simulink model "MyVhclOperator_RTW"  (Simulink 10.3)
settings: Solver=ode1  StartTime=0.0  StopTime=inf  FixedStep=0.001  RelTol=1e-3
PreLoadFcn:
  | vehicle = 'Car'; if ~length(which('cmcmd')), cmenv; end
  | MyVhclOperator_RTW_bus
InitFcn:
  | vehicle = 'Car'; if ~length(which('cmcmd')), cmenv; end
  | MyVhclOperator_RTW_bus
undefined symbols (not defined in the file or in its folder): OperationFinished, Phase, SteerAng, VCBus
libraries: simulink x45
(part 3 of 3)

== system MyVhclOperator_RTW/MyVhclOperator/Trg: OperState_Absent/OperState_Driving/Drive2Off/Wait until Standstill ==
  BusIn : Inport
  Action Port : ActionPort  ActionPortLabel=case: { }
  Bus Assignment : BusAssignment  AssignedSignals=Phase
  Bus Selector : BusSelector  OutputSignals=Velocity
  Compare To Constant : simulink/Logic and Bit Operations/Compare To Constant  SystemSampleTime=-1  relop=<=  const=0.1  LogicOutDataTypeMode=uint8
  Constant : Constant  Value=3
  Constant1 : Constant  Value=2
  Signal Conversion : SignalConversion  ConversionOutput=Bus copy  OverrideOpt=off
  Switch : Switch  Criteria=u2 ~= 0
  BusOut : Outport  InitialOutput=[0]  VectorParamsAs1DForOutWhenUnconnected=off
  wires:
  Bus Assignment/1 -> BusOut/1
  BusIn/1 -> Bus Selector/1, Signal Conversion/1
  Switch/1 -> Bus Assignment/2
  Bus Selector/1 -> Compare To Constant/1  "<Velocity>"
  Constant/1 -> Switch/1
  Constant1/1 -> Switch/3
  Compare To Constant/1 -> Switch/2
  Signal Conversion/1 -> Bus Assignment/1

== system MyVhclOperator_RTW/MyVhclOperator/Trg: OperState_Accessory/OperState_Driving/Drive2Off/Active Brake ==
  BusIn : Inport
  Action Port : ActionPort  ActionPortLabel=case: { }
  Bus Assignment1 : BusAssignment  AssignedSignals=VCBus.Key,VCBus.GearNo,VCBus.SelectorCtrl,VCBus.Gas,VCBus.Clutch,VCBus.Brake,VCBus.BrakePark,Phase
  Bus Selector : BusSelector  OutputSignals=GBKind
  Bus Selector1 : BusSelector  OutputSignals=Key,GearNo,SelectorCtrl,Gas,Clutch,Brake,BrakePark
  Constant : Constant  Value=2
  OperState: Braking : Subsystem
  Signal Conversion : SignalConversion  ConversionOutput=Bus copy  OverrideOpt=off
  BusOut : Outport  InitialOutput=[0]  VectorParamsAs1DForOutWhenUnconnected=off
  wires:
  BusIn/1 -> Bus Selector/1, Signal Conversion/1
  Bus Selector/1 -> OperState: Braking/1(GBKind)  "<GBKind>"
  OperState: Braking/1(BusOut) -> Bus Selector1/1  "VC_Bus"
  Constant/1 -> Bus Assignment1/9
  Bus Assignment1/1 -> BusOut/1
  Signal Conversion/1 -> Bus Assignment1/1
  Bus Selector1/1 -> Bus Assignment1/2  "<Key>"
  Bus Selector1/2 -> Bus Assignment1/3  "<GearNo>"
  Bus Selector1/3 -> Bus Assignment1/4  "<SelectorCtrl>"
  Bus Selector1/4 -> Bus Assignment1/5  "<Gas>"
  Bus Selector1/5 -> Bus Assignment1/6  "<Clutch>"
  Bus Selector1/6 -> Bus Assignment1/7  "<Brake>"
  Bus Selector1/7 -> Bus Assignment1/8  "<BrakePark>"

== system MyVhclOperator_RTW/MyVhclOperator/Trg: OperState_Accessory/OperState_Driving/Drive2Off/Brake to standstill? ==
  BusIn : Inport
  Action Port : ActionPort  ActionPortLabel=case: { }
  Bus Assignment : BusAssignment  AssignedSignals=Phase
  Bus Selector : BusSelector  OutputSignals=Velocity
  Compare To Constant : simulink/Logic and Bit Operations/Compare To Constant  SystemSampleTime=-1  relop=>  const=0.1  LogicOutDataTypeMode=uint8
  Constant : Constant
  Constant1 : Constant  Value=3
  Signal Conversion : SignalConversion  ConversionOutput=Bus copy  OverrideOpt=off
  Switch : Switch  Criteria=u2 ~= 0
  BusOut : Outport  InitialOutput=[0]  VectorParamsAs1DForOutWhenUnconnected=off
  wires:
  Bus Assignment/1 -> BusOut/1
  BusIn/1 -> Bus Selector/1, Signal Conversion/1
  Switch/1 -> Bus Assignment/2
  Bus Selector/1 -> Compare To Constant/1  "<Velocity>"
  Constant/1 -> Switch/1
  Constant1/1 -> Switch/3
  Compare To Constant/1 -> Switch/2
  Signal Conversion/1 -> Bus Assignment/1

== system MyVhclOperator_RTW/MyVhclOperator/Trg: OperState_Accessory/OperState_Driving/Drive2Off/Key PowerOff ==
  BusIn : Inport
  Action Port : ActionPort  ActionPortLabel=case: { }
  Bus Assignment : BusAssignment  AssignedSignals=VCBus.Key,SteerAng,Phase
  Constant : Constant  Value=4
  Constant2 : Constant  Value=0.0
  KeyPos_KeyIn_PowerOff : Constant
  Signal Conversion : SignalConversion  ConversionOutput=Bus copy  OverrideOpt=off
  BusOut : Outport  InitialOutput=[0]  VectorParamsAs1DForOutWhenUnconnected=off
  wires:
  BusIn/1 -> Signal Conversion/1
  Bus Assignment/1 -> BusOut/1
  Constant/1 -> Bus Assignment/4
  Constant2/1 -> Bus Assignment/3
  KeyPos_KeyIn_PowerOff/1 -> Bus Assignment/2
  Signal Conversion/1 -> Bus Assignment/1

== system MyVhclOperator_RTW/MyVhclOperator/Trg: OperState_Accessory/OperState_Driving/Drive2Off/Wait for PowerOff ==
  BusIn : Inport
  Action Port : ActionPort  ActionPortLabel=case: { }
  Signal Conversion : SignalConversion  ConversionOutput=Bus copy  OverrideOpt=off
  BusOut : Outport  VectorParamsAs1DForOutWhenUnconnected=off
  wires:
  BusIn/1 -> Signal Conversion/1
  Signal Conversion/1 -> BusOut/1

== system MyVhclOperator_RTW/MyVhclOperator/Trg: OperState_Accessory/OperState_Driving/Drive2Off/Wait until Standstill ==
  BusIn : Inport
  Action Port : ActionPort  ActionPortLabel=case: { }
  Bus Assignment : BusAssignment  AssignedSignals=Phase
  Bus Selector : BusSelector  OutputSignals=Velocity
  Compare To Constant : simulink/Logic and Bit Operations/Compare To Constant  SystemSampleTime=-1  relop=<=  const=0.1  LogicOutDataTypeMode=uint8
  Constant : Constant  Value=3
  Constant1 : Constant  Value=2
  Signal Conversion : SignalConversion  ConversionOutput=Bus copy  OverrideOpt=off
  Switch : Switch  Criteria=u2 ~= 0
  BusOut : Outport  InitialOutput=[0]  VectorParamsAs1DForOutWhenUnconnected=off
  wires:
  Bus Assignment/1 -> BusOut/1
  BusIn/1 -> Bus Selector/1, Signal Conversion/1
  Switch/1 -> Bus Assignment/2
  Bus Selector/1 -> Compare To Constant/1  "<Velocity>"
  Constant/1 -> Switch/1
  Constant1/1 -> Switch/3
  Compare To Constant/1 -> Switch/2
  Signal Conversion/1 -> Bus Assignment/1

== system MyVhclOperator_RTW/MyVhclOperator/Trg: OperState_PowerOff/OperState_Driving/Drive2Off/Active Brake ==
  BusIn : Inport
  Action Port : ActionPort  ActionPortLabel=case: { }
  Bus Assignment1 : BusAssignment  AssignedSignals=VCBus.Key,VCBus.GearNo,VCBus.SelectorCtrl,VCBus.Gas,VCBus.Clutch,VCBus.Brake,VCBus.BrakePark,Phase
  Bus Selector : BusSelector  OutputSignals=GBKind
  Bus Selector1 : BusSelector  OutputSignals=Key,GearNo,SelectorCtrl,Gas,Clutch,Brake,BrakePark
  Constant : Constant  Value=2
  OperState: Braking : Subsystem
  Signal Conversion : SignalConversion  ConversionOutput=Bus copy  OverrideOpt=off
  BusOut : Outport  InitialOutput=[0]  VectorParamsAs1DForOutWhenUnconnected=off
  wires:
  BusIn/1 -> Bus Selector/1, Signal Conversion/1
  Bus Selector/1 -> OperState: Braking/1(GBKind)  "<GBKind>"
  OperState: Braking/1(BusOut) -> Bus Selector1/1  "VC_Bus"
  Constant/1 -> Bus Assignment1/9
  Bus Assignment1/1 -> BusOut/1
  Signal Conversion/1 -> Bus Assignment1/1
  Bus Selector1/1 -> Bus Assignment1/2  "<Key>"
  Bus Selector1/2 -> Bus Assignment1/3  "<GearNo>"
  Bus Selector1/3 -> Bus Assignment1/4  "<SelectorCtrl>"
  Bus Selector1/4 -> Bus Assignment1/5  "<Gas>"
  Bus Selector1/5 -> Bus Assignment1/6  "<Clutch>"
  Bus Selector1/6 -> Bus Assignment1/7  "<Brake>"
  Bus Selector1/7 -> Bus Assignment1/8  "<BrakePark>"

== system MyVhclOperator_RTW/MyVhclOperator/Trg: OperState_PowerOff/OperState_Driving/Drive2Off/Brake to standstill? ==
  BusIn : Inport
  Action Port : ActionPort  ActionPortLabel=case: { }
  Bus Assignment : BusAssignment  AssignedSignals=Phase
  Bus Selector : BusSelector  OutputSignals=Velocity
  Compare To Constant : simulink/Logic and Bit Operations/Compare To Constant  SystemSampleTime=-1  relop=>  const=0.1  LogicOutDataTypeMode=uint8
  Constant : Constant
  Constant1 : Constant  Value=3
  Signal Conversion : SignalConversion  ConversionOutput=Bus copy  OverrideOpt=off
  Switch : Switch  Criteria=u2 ~= 0
  BusOut : Outport  InitialOutput=[0]  VectorParamsAs1DForOutWhenUnconnected=off
  wires:
  Bus Assignment/1 -> BusOut/1
  BusIn/1 -> Bus Selector/1, Signal Conversion/1
  Switch/1 -> Bus Assignment/2
  Bus Selector/1 -> Compare To Constant/1  "<Velocity>"
  Constant/1 -> Switch/1
  Constant1/1 -> Switch/3
  Compare To Constant/1 -> Switch/2
  Signal Conversion/1 -> Bus Assignment/1

== system MyVhclOperator_RTW/MyVhclOperator/Trg: OperState_PowerOff/OperState_Driving/Drive2Off/Key PowerOff ==
  BusIn : Inport
  Action Port : ActionPort  ActionPortLabel=case: { }
  Bus Assignment : BusAssignment  AssignedSignals=VCBus.Key,SteerAng,Phase
  Constant : Constant  Value=4
  Constant2 : Constant  Value=0.0
  KeyPos_KeyIn_PowerOff : Constant
  Signal Conversion : SignalConversion  ConversionOutput=Bus copy  OverrideOpt=off
  BusOut : Outport  InitialOutput=[0]  VectorParamsAs1DForOutWhenUnconnected=off
  wires:
  BusIn/1 -> Signal Conversion/1
  Bus Assignment/1 -> BusOut/1
  Constant/1 -> Bus Assignment/4
  Constant2/1 -> Bus Assignment/3
  KeyPos_KeyIn_PowerOff/1 -> Bus Assignment/2
  Signal Conversion/1 -> Bus Assignment/1

== system MyVhclOperator_RTW/MyVhclOperator/Trg: OperState_PowerOff/OperState_Driving/Drive2Off/Wait for PowerOff ==
  BusIn : Inport
  Action Port : ActionPort  ActionPortLabel=case: { }
  Signal Conversion : SignalConversion  ConversionOutput=Bus copy  OverrideOpt=off
  BusOut : Outport  VectorParamsAs1DForOutWhenUnconnected=off
  wires:
  BusIn/1 -> Signal Conversion/1
  Signal Conversion/1 -> BusOut/1

== system MyVhclOperator_RTW/MyVhclOperator/Trg: OperState_PowerOff/OperState_Driving/Drive2Off/Wait until Standstill ==
  BusIn : Inport
  Action Port : ActionPort  ActionPortLabel=case: { }
  Bus Assignment : BusAssignment  AssignedSignals=Phase
  Bus Selector : BusSelector  OutputSignals=Velocity
  Compare To Constant : simulink/Logic and Bit Operations/Compare To Constant  SystemSampleTime=-1  relop=<=  const=0.1  LogicOutDataTypeMode=uint8
  Constant : Constant  Value=3
  Constant1 : Constant  Value=2
  Signal Conversion : SignalConversion  ConversionOutput=Bus copy  OverrideOpt=off
  Switch : Switch  Criteria=u2 ~= 0
  BusOut : Outport  InitialOutput=[0]  VectorParamsAs1DForOutWhenUnconnected=off
  wires:
  Bus Assignment/1 -> BusOut/1
  BusIn/1 -> Bus Selector/1, Signal Conversion/1
  Switch/1 -> Bus Assignment/2
  Bus Selector/1 -> Compare To Constant/1  "<Velocity>"
  Constant/1 -> Switch/1
  Constant1/1 -> Switch/3
  Compare To Constant/1 -> Switch/2
  Signal Conversion/1 -> Bus Assignment/1

== system MyVhclOperator_RTW/MyVhclOperator/Trg: OperState_PowerOn/OperState_Driving/Drive2Off/Active Brake ==
  BusIn : Inport
  Action Port : ActionPort  ActionPortLabel=case: { }
  Bus Assignment1 : BusAssignment  AssignedSignals=VCBus.Key,VCBus.GearNo,VCBus.SelectorCtrl,VCBus.Gas,VCBus.Clutch,VCBus.Brake,VCBus.BrakePark,Phase
  Bus Selector : BusSelector  OutputSignals=GBKind
  Bus Selector1 : BusSelector  OutputSignals=Key,GearNo,SelectorCtrl,Gas,Clutch,Brake,BrakePark
  Constant : Constant  Value=2
  OperState: Braking : Subsystem
  Signal Conversion : SignalConversion  ConversionOutput=Bus copy  OverrideOpt=off
  BusOut : Outport  InitialOutput=[0]  VectorParamsAs1DForOutWhenUnconnected=off
  wires:
  BusIn/1 -> Bus Selector/1, Signal Conversion/1
  Bus Selector/1 -> OperState: Braking/1(GBKind)  "<GBKind>"
  OperState: Braking/1(BusOut) -> Bus Selector1/1  "VC_Bus"
  Constant/1 -> Bus Assignment1/9
  Bus Assignment1/1 -> BusOut/1
  Signal Conversion/1 -> Bus Assignment1/1
  Bus Selector1/1 -> Bus Assignment1/2  "<Key>"
  Bus Selector1/2 -> Bus Assignment1/3  "<GearNo>"
  Bus Selector1/3 -> Bus Assignment1/4  "<SelectorCtrl>"
  Bus Selector1/4 -> Bus Assignment1/5  "<Gas>"
  Bus Selector1/5 -> Bus Assignment1/6  "<Clutch>"
  Bus Selector1/6 -> Bus Assignment1/7  "<Brake>"
  Bus Selector1/7 -> Bus Assignment1/8  "<BrakePark>"

== system MyVhclOperator_RTW/MyVhclOperator/Trg: OperState_PowerOn/OperState_Driving/Drive2Off/Brake to standstill? ==
  BusIn : Inport
  Action Port : ActionPort  ActionPortLabel=case: { }
  Bus Assignment : BusAssignment  AssignedSignals=Phase
  Bus Selector : BusSelector  OutputSignals=Velocity
  Compare To Constant : simulink/Logic and Bit Operations/Compare To Constant  SystemSampleTime=-1  relop=>  const=0.1  LogicOutDataTypeMode=uint8
  Constant : Constant
  Constant1 : Constant  Value=3
  Signal Conversion : SignalConversion  ConversionOutput=Bus copy  OverrideOpt=off
  Switch : Switch  Criteria=u2 ~= 0
  BusOut : Outport  InitialOutput=[0]  VectorParamsAs1DForOutWhenUnconnected=off
  wires:
  Bus Assignment/1 -> BusOut/1
  BusIn/1 -> Bus Selector/1, Signal Conversion/1
  Switch/1 -> Bus Assignment/2
  Bus Selector/1 -> Compare To Constant/1  "<Velocity>"
  Constant/1 -> Switch/1
  Constant1/1 -> Switch/3
  Compare To Constant/1 -> Switch/2
  Signal Conversion/1 -> Bus Assignment/1

== system MyVhclOperator_RTW/MyVhclOperator/Trg: OperState_PowerOn/OperState_Driving/Drive2Off/Key PowerOff ==
  BusIn : Inport
  Action Port : ActionPort  ActionPortLabel=case: { }
  Bus Assignment : BusAssignment  AssignedSignals=VCBus.Key,SteerAng,Phase
  Constant : Constant  Value=4
  Constant2 : Constant  Value=0.0
  KeyPos_KeyIn_PowerOff : Constant
  Signal Conversion : SignalConversion  ConversionOutput=Bus copy  OverrideOpt=off
  BusOut : Outport  InitialOutput=[0]  VectorParamsAs1DForOutWhenUnconnected=off
  wires:
  BusIn/1 -> Signal Conversion/1
  Bus Assignment/1 -> BusOut/1
  Constant/1 -> Bus Assignment/4
  Constant2/1 -> Bus Assignment/3
  KeyPos_KeyIn_PowerOff/1 -> Bus Assignment/2
  Signal Conversion/1 -> Bus Assignment/1

== system MyVhclOperator_RTW/MyVhclOperator/Trg: OperState_PowerOn/OperState_Driving/Drive2Off/Wait for PowerOff ==
  BusIn : Inport
  Action Port : ActionPort  ActionPortLabel=case: { }
  Signal Conversion : SignalConversion  ConversionOutput=Bus copy  OverrideOpt=off
  BusOut : Outport  VectorParamsAs1DForOutWhenUnconnected=off
  wires:
  BusIn/1 -> Signal Conversion/1
  Signal Conversion/1 -> BusOut/1

== system MyVhclOperator_RTW/MyVhclOperator/Trg: OperState_PowerOn/OperState_Driving/Drive2Off/Wait until Standstill ==
  BusIn : Inport
  Action Port : ActionPort  ActionPortLabel=case: { }
  Bus Assignment : BusAssignment  AssignedSignals=Phase
  Bus Selector : BusSelector  OutputSignals=Velocity
  Compare To Constant : simulink/Logic and Bit Operations/Compare To Constant  SystemSampleTime=-1  relop=<=  const=0.1  LogicOutDataTypeMode=uint8
  Constant : Constant  Value=3
  Constant1 : Constant  Value=2
  Signal Conversion : SignalConversion  ConversionOutput=Bus copy  OverrideOpt=off
  Switch : Switch  Criteria=u2 ~= 0
  BusOut : Outport  InitialOutput=[0]  VectorParamsAs1DForOutWhenUnconnected=off
  wires:
  Bus Assignment/1 -> BusOut/1
  BusIn/1 -> Bus Selector/1, Signal Conversion/1
  Switch/1 -> Bus Assignment/2
  Bus Selector/1 -> Compare To Constant/1  "<Velocity>"
  Constant/1 -> Switch/1
  Constant1/1 -> Switch/3
  Compare To Constant/1 -> Switch/2
  Signal Conversion/1 -> Bus Assignment/1

== system MyVhclOperator_RTW/MyVhclOperator/Trg: OperState_Absent/OperState_Driving/Drive2Off/Active Brake/OperState: Braking ==
  note: Operation State:
      | Braking
  GBKind : Inport
  Brake : Constant  Value=0.6
  BrakePark : Constant  Value=0.0
  Bus Creator : BusCreator  Inputs=7
  Bus Creator1 : BusCreator  Inputs=3
  Bus Creator2 : BusCreator  Inputs=3
  Bus Selector : BusSelector  OutputSignals=GearNo,Clutch,SelectorCtrl
  Clutch : Constant  Value=1.0
  GBKind_Manual : simulink/Logic and Bit Operations/Compare To Constant  SystemSampleTime=-1  relop===  const=1  LogicOutDataTypeMode=uint8
  Gas : Constant  Value=0.0
  GearNo : Constant  Value=0
  KeyPos_KeyOut : Constant  Value=3
  No_Clutch : Constant  Value=0.0
  No_GearNo : Constant  Value=0
  No_SelectorCtrl : Constant  Value=0
  SelectorCtrl_P : Constant  Value=0
  Switch : Switch  Criteria=u2 ~= 0
  BusOut : Outport  VectorParamsAs1DForOutWhenUnconnected=off
  wires:
  GBKind_Manual/1 -> Switch/2
  GBKind/1 -> GBKind_Manual/1
  Bus Creator2/1 -> Switch/3
  SelectorCtrl_P/1 -> Bus Creator2/3  "SelectorCtrl"
  No_Clutch/1 -> Bus Creator2/2  "Clutch"
  No_GearNo/1 -> Bus Creator2/1  "GearNo"
  No_SelectorCtrl/1 -> Bus Creator1/3  "SelectorCtrl"
  Clutch/1 -> Bus Creator1/2  "Clutch"
  GearNo/1 -> Bus Creator1/1  "GearNo"
  Bus Creator1/1 -> Switch/1
  Switch/1 -> Bus Selector/1
  BrakePark/1 -> Bus Creator/7  "BrakePark"
  Brake/1 -> Bus Creator/6  "Brake"
  Gas/1 -> Bus Creator/5  "Gas"
  KeyPos_KeyOut/1 -> Bus Creator/4  "Key"
  Bus Selector/3 -> Bus Creator/3  "<SelectorCtrl>"
  Bus Selector/2 -> Bus Creator/2  "<Clutch>"
  Bus Selector/1 -> Bus Creator/1  "<GearNo>"
  Bus Creator/1 -> BusOut/1

== system MyVhclOperator_RTW/MyVhclOperator/Trg: OperState_Accessory/OperState_Driving/Drive2Off/Active Brake/OperState: Braking ==
  note: Operation State:
      | Braking
  GBKind : Inport
  Brake : Constant  Value=0.6
  BrakePark : Constant  Value=0.0
  Bus Creator : BusCreator  Inputs=7
  Bus Creator1 : BusCreator  Inputs=3
  Bus Creator2 : BusCreator  Inputs=3
  Bus Selector : BusSelector  OutputSignals=GearNo,Clutch,SelectorCtrl
  Clutch : Constant  Value=1.0
  GBKind_Manual : simulink/Logic and Bit Operations/Compare To Constant  SystemSampleTime=-1  relop===  const=1  LogicOutDataTypeMode=uint8
  Gas : Constant  Value=0.0
  GearNo : Constant  Value=0
  KeyPos_KeyOut : Constant  Value=3
  No_Clutch : Constant  Value=0.0
  No_GearNo : Constant  Value=0
  No_SelectorCtrl : Constant  Value=0
  SelectorCtrl_P : Constant  Value=0
  Switch : Switch  Criteria=u2 ~= 0
  BusOut : Outport  VectorParamsAs1DForOutWhenUnconnected=off
  wires:
  GBKind_Manual/1 -> Switch/2
  GBKind/1 -> GBKind_Manual/1
  Bus Creator2/1 -> Switch/3
  SelectorCtrl_P/1 -> Bus Creator2/3  "SelectorCtrl"
  No_Clutch/1 -> Bus Creator2/2  "Clutch"
  No_GearNo/1 -> Bus Creator2/1  "GearNo"
  No_SelectorCtrl/1 -> Bus Creator1/3  "SelectorCtrl"
  Clutch/1 -> Bus Creator1/2  "Clutch"
  GearNo/1 -> Bus Creator1/1  "GearNo"
  Bus Creator1/1 -> Switch/1
  Switch/1 -> Bus Selector/1
  BrakePark/1 -> Bus Creator/7  "BrakePark"
  Brake/1 -> Bus Creator/6  "Brake"
  Gas/1 -> Bus Creator/5  "Gas"
  KeyPos_KeyOut/1 -> Bus Creator/4  "Key"
  Bus Selector/3 -> Bus Creator/3  "<SelectorCtrl>"
  Bus Selector/2 -> Bus Creator/2  "<Clutch>"
  Bus Selector/1 -> Bus Creator/1  "<GearNo>"
  Bus Creator/1 -> BusOut/1

== system MyVhclOperator_RTW/MyVhclOperator/Trg: OperState_PowerOff/OperState_Driving/Drive2Off/Active Brake/OperState: Braking ==
  note: Operation State:
      | Braking
  GBKind : Inport
  Brake : Constant  Value=0.6
  BrakePark : Constant  Value=0.0
  Bus Creator : BusCreator  Inputs=7
  Bus Creator1 : BusCreator  Inputs=3
  Bus Creator2 : BusCreator  Inputs=3
  Bus Selector : BusSelector  OutputSignals=GearNo,Clutch,SelectorCtrl
  Clutch : Constant  Value=1.0
  GBKind_Manual : simulink/Logic and Bit Operations/Compare To Constant  SystemSampleTime=-1  relop===  const=1  LogicOutDataTypeMode=uint8
  Gas : Constant  Value=0.0
  GearNo : Constant  Value=0
  KeyPos_KeyOut : Constant  Value=3
  No_Clutch : Constant  Value=0.0
  No_GearNo : Constant  Value=0
  No_SelectorCtrl : Constant  Value=0
  SelectorCtrl_P : Constant  Value=0
  Switch : Switch  Criteria=u2 ~= 0
  BusOut : Outport  VectorParamsAs1DForOutWhenUnconnected=off
  wires:
  GBKind_Manual/1 -> Switch/2
  GBKind/1 -> GBKind_Manual/1
  Bus Creator2/1 -> Switch/3
  SelectorCtrl_P/1 -> Bus Creator2/3  "SelectorCtrl"
  No_Clutch/1 -> Bus Creator2/2  "Clutch"
  No_GearNo/1 -> Bus Creator2/1  "GearNo"
  No_SelectorCtrl/1 -> Bus Creator1/3  "SelectorCtrl"
  Clutch/1 -> Bus Creator1/2  "Clutch"
  GearNo/1 -> Bus Creator1/1  "GearNo"
  Bus Creator1/1 -> Switch/1
  Switch/1 -> Bus Selector/1
  BrakePark/1 -> Bus Creator/7  "BrakePark"
  Brake/1 -> Bus Creator/6  "Brake"
  Gas/1 -> Bus Creator/5  "Gas"
  KeyPos_KeyOut/1 -> Bus Creator/4  "Key"
  Bus Selector/3 -> Bus Creator/3  "<SelectorCtrl>"
  Bus Selector/2 -> Bus Creator/2  "<Clutch>"
  Bus Selector/1 -> Bus Creator/1  "<GearNo>"
  Bus Creator/1 -> BusOut/1

== system MyVhclOperator_RTW/MyVhclOperator/Trg: OperState_PowerOn/OperState_Driving/Drive2Off/Active Brake/OperState: Braking ==
  note: Operation State:
      | Braking
  GBKind : Inport
  Brake : Constant  Value=0.6
  BrakePark : Constant  Value=0.0
  Bus Creator : BusCreator  Inputs=7
  Bus Creator1 : BusCreator  Inputs=3
  Bus Creator2 : BusCreator  Inputs=3
  Bus Selector : BusSelector  OutputSignals=GearNo,Clutch,SelectorCtrl
  Clutch : Constant  Value=1.0
  GBKind_Manual : simulink/Logic and Bit Operations/Compare To Constant  SystemSampleTime=-1  relop===  const=1  LogicOutDataTypeMode=uint8
  Gas : Constant  Value=0.0
  GearNo : Constant  Value=0
  KeyPos_KeyOut : Constant  Value=3
  No_Clutch : Constant  Value=0.0
  No_GearNo : Constant  Value=0
  No_SelectorCtrl : Constant  Value=0
  SelectorCtrl_P : Constant  Value=0
  Switch : Switch  Criteria=u2 ~= 0
  BusOut : Outport  VectorParamsAs1DForOutWhenUnconnected=off
  wires:
  GBKind_Manual/1 -> Switch/2
  GBKind/1 -> GBKind_Manual/1
  Bus Creator2/1 -> Switch/3
  SelectorCtrl_P/1 -> Bus Creator2/3  "SelectorCtrl"
  No_Clutch/1 -> Bus Creator2/2  "Clutch"
  No_GearNo/1 -> Bus Creator2/1  "GearNo"
  No_SelectorCtrl/1 -> Bus Creator1/3  "SelectorCtrl"
  Clutch/1 -> Bus Creator1/2  "Clutch"
  GearNo/1 -> Bus Creator1/1  "GearNo"
  Bus Creator1/1 -> Switch/1
  Switch/1 -> Bus Selector/1
  BrakePark/1 -> Bus Creator/7  "BrakePark"
  Brake/1 -> Bus Creator/6  "Brake"
  Gas/1 -> Bus Creator/5  "Gas"
  KeyPos_KeyOut/1 -> Bus Creator/4  "Key"
  Bus Selector/3 -> Bus Creator/3  "<SelectorCtrl>"
  Bus Selector/2 -> Bus Creator/2  "<Clutch>"
  Bus Selector/1 -> Bus Creator/1  "<GearNo>"
  Bus Creator/1 -> BusOut/1
